simulink model "Dynamic_Control"  (R2015b)
settings: Solver=FixedStepAuto  StartTime=0  StopTime=26  FixedStep=0.1  RelTol=1e-3
values from neighbouring files (symbols this model uses):
  Kd = 8    [init.m]
  Kp = 8    [init.m]
  L = 0.13    [init.m]
  r = 0.1    [init.m]
  R = 2    [init.m]
  Theta0 = pi    (= 3.14159265359)    [init.m]
  wd = 0.5    [init.m]
  X0 = 2.3    [init.m]
  Y0 = 0    [init.m]
undefined symbols (not defined in the file): alpha, d
libraries: simulink x2
settings Model: Creator=GANESH  LastModifiedBy=GANESH
settings SolverCC: AlgebraicLoopSolver=LineSearch

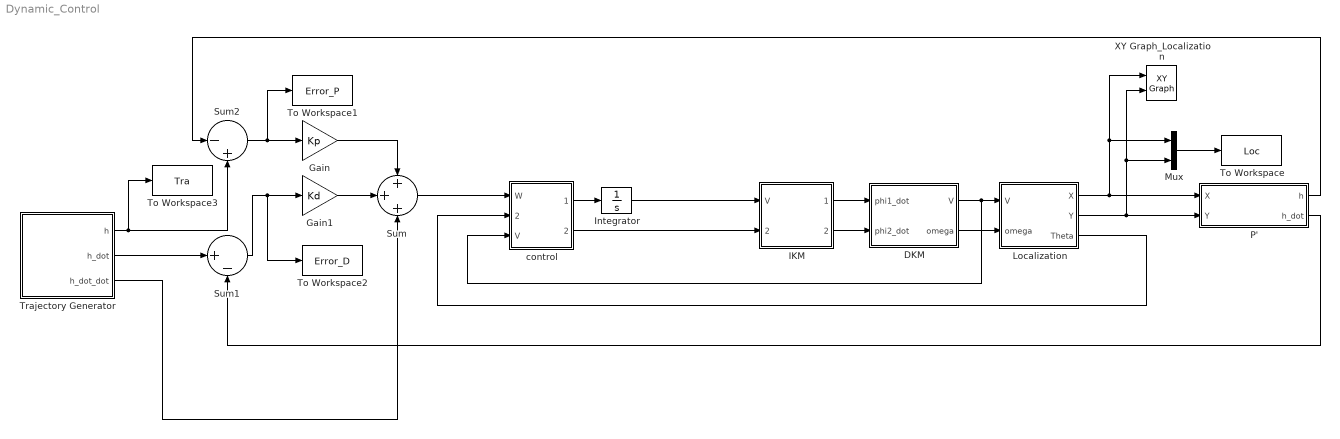
== system Dynamic_Control ==
  DKM : Subsystem  mask{r=r, L=L}
      mask prompts: r "Radius of the wheel"; L "Half of the wheelbase"
  Gain : Gain  Gain=Kp
  Gain1 : Gain  Gain=Kd
  IKM : Subsystem  mask{r=(1+alpha)*r, L=(1+alpha)*L}
      mask prompts: r "Radius of wheel (estimated)"; L "Half of wheelbase (estimated)"
  Integrator : Integrator  InitialCondition=1.2
  Localization : Subsystem
  Mux : Mux  Inputs=2
  P' : Subsystem  mask{d=d}
      mask prompts: d "Position of point on robot"
  Sum : Sum  Inputs=+++
  Sum1 : Sum  Inputs=|+-
  Sum2 : Sum  Inputs=|-+
  To Workspace : ToWorkspace  VariableName=Loc  SaveFormat=Timeseries  SampleTime=-1
  To Workspace1 : ToWorkspace  VariableName=Error_P  SaveFormat=Timeseries  SampleTime=-1
  To Workspace2 : ToWorkspace  VariableName=Error_D  SaveFormat=Timeseries  SampleTime=-1
  To Workspace3 : ToWorkspace  VariableName=Tra  SaveFormat=Timeseries  SampleTime=-1
  Trajectory Generator : Subsystem  mask{R=R, wd=wd}
      mask prompts: R "Radius of Circular Trajectory"; wd "Desired Angular Velocity"
  XY Graph_Localization : simulink/Sinks/XY Graph  xmin=-5  xmax=5  ymin=-5  ymax=5  st=-1
  control : Subsystem  mask{rp=d}
      mask prompts: rp "Distance of point on robot"
  wires:
  Sum1/1 -> To Workspace2/1, Gain1/1
  Sum2/1 -> To Workspace1/1, Gain/1
  control/1(V_dot) -> Integrator/1
  P'/1(h) -> Sum2/1
  P'/2(h_dot) -> Sum1/2
  Gain1/1 -> Sum/2
  Gain/1 -> Sum/1
  Trajectory Generator/3(h_dot_dot) -> Sum/3
  Sum/1 -> control/1(W)
  Localization/1(X) -> P'/1(X), XY Graph_Localization/1, Mux/1
  IKM/1(phi1_dot) -> DKM/1(phi1_dot)
  IKM/2(phi2_dot) -> DKM/2(phi2_dot)
  Localization/2(Y) -> P'/2(Y), Mux/2, XY Graph_Localization/2
  Localization/3(Theta) -> control/2(Theta)
  Trajectory Generator/1(h) -> To Workspace3/1, Sum2/2
  Trajectory Generator/2(h_dot) -> Sum1/1
  Integrator/1 -> IKM/1(V)
  DKM/1(V) -> control/3(V), Localization/1(V)
  DKM/2(omega) -> Localization/2(omega)
  control/2(omega) -> IKM/2(omega)
  Mux/1 -> To Workspace/1

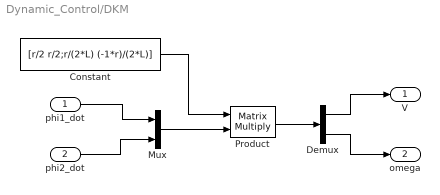
== system Dynamic_Control/DKM ==
  phi1_dot : Inport
  phi2_dot : Inport  Port=2
  Constant : Constant  Value=[r/2 r/2;r/(2*L) (-1*r)/(2*L)]
  Demux : Demux  Outputs=2
  Mux : Mux  Inputs=2
  Product : Product  Multiplication=Matrix(*)
  V : Outport
  omega : Outport  Port=2
  wires:
  Product/1 -> Demux/1
  phi1_dot/1 -> Mux/1
  Demux/1 -> V/1
  phi2_dot/1 -> Mux/2
  Constant/1 -> Product/1
  Demux/2 -> omega/1
  Mux/1 -> Product/2

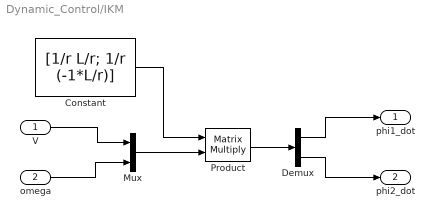
== system Dynamic_Control/IKM ==
  V : Inport
  omega : Inport  Port=2
  Constant : Constant  Value=[1/r L/r; 1/r (-1*L/r)]
  Demux : Demux  Outputs=2
  Mux : Mux  Inputs=2
  Product : Product  Multiplication=Matrix(*)
  phi1_dot : Outport
  phi2_dot : Outport  Port=2
  wires:
  Product/1 -> Demux/1
  V/1 -> Mux/1
  Demux/1 -> phi1_dot/1
  omega/1 -> Mux/2
  Constant/1 -> Product/1
  Mux/1 -> Product/2
  Demux/2 -> phi2_dot/1

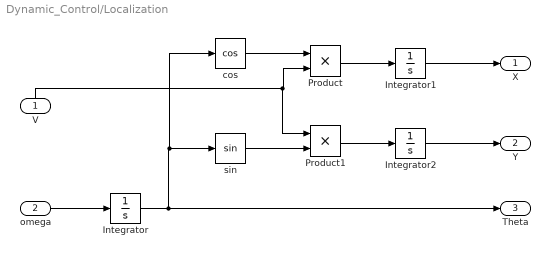
== system Dynamic_Control/Localization ==
  V : Inport
  omega : Inport  Port=2
  Integrator : Integrator  InitialCondition=Theta0
  Integrator1 : Integrator  InitialCondition=X0
  Integrator2 : Integrator  InitialCondition=Y0
  Product : Product
  Product1 : Product
  cos : Trigonometry  Operator=cos
  sin : Trigonometry
  X : Outport
  Y : Outport  Port=2
  Theta : Outport  Port=3
  wires:
  Integrator/1 -> Theta/1, cos/1, sin/1
  V/1 -> Product1/1, Product/2
  omega/1 -> Integrator/1
  cos/1 -> Product/1
  sin/1 -> Product1/2
  Integrator1/1 -> X/1
  Product1/1 -> Integrator2/1
  Integrator2/1 -> Y/1
  Product/1 -> Integrator1/1

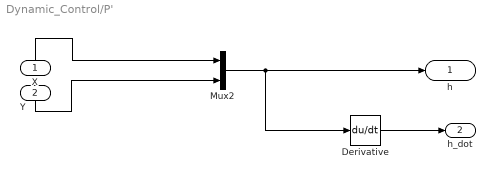
== system Dynamic_Control/P' ==
  X : Inport
  Y : Inport  Port=2
  Derivative : Derivative
  Mux2 : Mux  Inputs=2
  h : Outport
  h_dot : Outport  Port=2
  wires:
  Y/1 -> Mux2/2
  X/1 -> Mux2/1
  Mux2/1 -> Derivative/1, h/1
  Derivative/1 -> h_dot/1

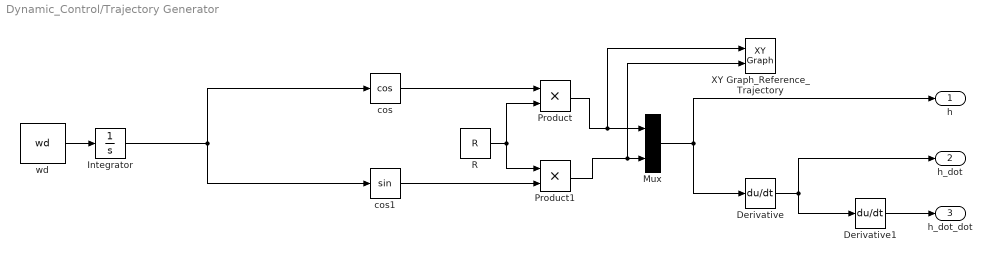
== system Dynamic_Control/Trajectory Generator ==
  Derivative : Derivative
  Derivative1 : Derivative
  Integrator : Integrator
  Mux : Mux  Inputs=2
  Product : Product
  Product1 : Product
  R : Constant  Value=R
  XY Graph_Reference_Trajectory : simulink/Sinks/XY Graph  xmin=-5  xmax=5  ymin=-5  ymax=5  st=-1
  cos : Trigonometry  Operator=cos
  cos1 : Trigonometry
  wd : Constant  Value=wd
  h : Outport
  h_dot : Outport  Port=2
  h_dot_dot : Outport  Port=3
  wires:
  R/1 -> Product/2, Product1/1
  Product1/1 -> XY Graph_Reference_Trajectory/2, Mux/2
  Product/1 -> Mux/1, XY Graph_Reference_Trajectory/1
  wd/1 -> Integrator/1
  Integrator/1 -> cos1/1, cos/1
  Mux/1 -> h/1, Derivative/1
  cos/1 -> Product/1
  cos1/1 -> Product1/2
  Derivative/1 -> h_dot/1, Derivative1/1
  Derivative1/1 -> h_dot_dot/1

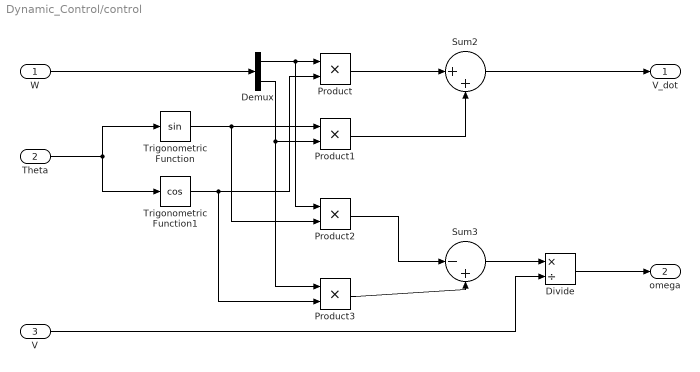
== system Dynamic_Control/control ==
  W : Inport
  Theta : Inport  Port=2
  V : Inport  Port=3
  Demux : Demux  Outputs=2
  Divide : Product  Inputs=*/
  Product{,1..3} (4 alike) : Product
  Sum2 : Sum  Inputs=|++
  Sum3 : Sum  Inputs=|-+
  Trigonometric Function : Trigonometry
  Trigonometric Function1 : Trigonometry  Operator=cos
  V_dot : Outport
  omega : Outport  Port=2
  wires:
  Product/1 -> Sum2/1
  Trigonometric Function1/1 -> Product3/2, Product/2
  Product3/1 -> Sum3/2
  Trigonometric Function/1 -> Product2/2, Product1/1
  Demux/1 -> Product2/1, Product/1
  Sum2/1 -> V_dot/1
  Product1/1 -> Sum2/2
  W/1 -> Demux/1
  Product2/1 -> Sum3/1
  Theta/1 -> Trigonometric Function1/1, Trigonometric Function/1
  Sum3/1 -> Divide/1
  Demux/2 -> Product3/1, Product1/2
  Divide/1 -> omega/1
  V/1 -> Divide/2
